simulink model "CT_transferfunctionProportionalDerivativecontroller_t1"  (R2015a)
settings: Solver=ode45  StartTime=0.0  StopTime=10.0  RelTol=1e-3
libraries: simulink x1
settings Model: Creator=Abu Bakar  LastModifiedBy=Abu Bakar

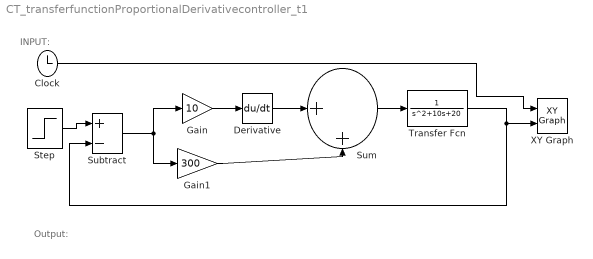
== system CT_transferfunctionProportionalDerivativecontroller_t1 ==
  note: Output:
  note: INPUT:
  Clock : Clock
  Derivative : Derivative
  Gain : Gain  Gain=10
  Gain1 : Gain  Gain=300
  Step : Step  SampleTime=0
  Subtract : Sum  Inputs=+-
  Sum : Sum  Inputs=|++
  Transfer Fcn : TransferFcn  Denominator=[1 10 20]  ContinuousStateAttributes='Position'
  XY Graph : simulink/Sinks/XY Graph  xmin=-1  xmax=10  ymin=-1  ymax=5  st=-1
  wires:
  Gain/1 -> Derivative/1
  Derivative/1 -> Sum/1
  Gain1/1 -> Sum/2
  Subtract/1 -> Gain/1, Gain1/1
  Step/1 -> Subtract/1
  Clock/1 -> XY Graph/1
  Sum/1 -> Transfer Fcn/1
  Transfer Fcn/1 -> Subtract/2, XY Graph/2
